simulink model "Roll_Pitch_LQIDG"  (R2020a)
settings: Solver=ode4  StartTime=0.0  StopTime=200  FixedStep=0.02  RelTol=1e-3
InitFcn:
  | LQIDG_solver;
values from neighbouring files (symbols this model uses):
  A1 = (h_cg * g * m_tot) / (m_tot * h_cg^2 + J_xx)    [QuadConstants.m]
  A3 = (b * d_cg) / (m_tot * h_cg^2 + J_xx)    [QuadConstants.m]
  A4 = (J_R) / (m_tot * h_cg^2 + J_xx)    [QuadConstants.m]
  A5 = (m1 * g * miu_k * r_x) / (m_tot * h_cg^2 + J_xx)    [QuadConstants.m]
  B3 = (b * d_cg) / (m_tot * h_cg^2 + J_yy)    [QuadConstants.m]
  LQIDG_openloop_pitch = (R1_inv * B' * p1)    [OpenLoop_LQDG_riccati_solver_pitch.m]
  LQIDG_openloop_roll = (R1_inv * B' * p1)    [OpenLoop_LQDG_riccati_solver_roll.m]
undefined symbols (not defined in the file or in its folder): A6, b, B6, d_cg, DiscIntNeverNeededParam, g, h_cg, J_R, J_yy, m2, m_tot, magnitude, miu_k, r_y
libraries: simulink x1, eeGeneralControl x1
settings Model: Creator=Ali  LastModifiedBy=Ali

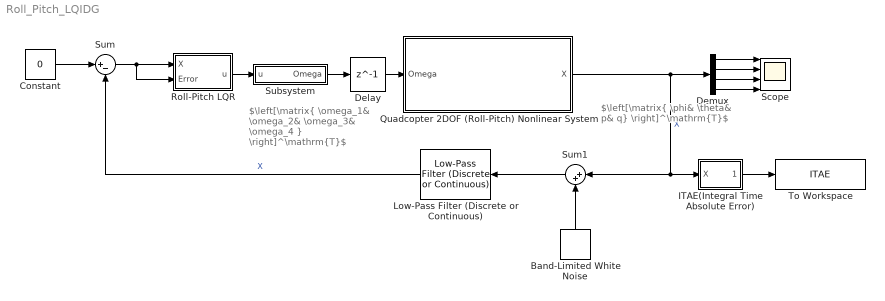
== system Roll_Pitch_LQIDG ==
  note: $\left[\matrix{ \omega_1& \omega_2& \omega_3& \omega_4 } \right]^\mathrm{T}$
  note: $\left[\matrix{ \phi& \theta& p& q} \right]^\mathrm{T}$
  Band-Limited White Noise : simulink/Sources/Band-Limited White Noise  Cov=[0.0001]  Ts=0.02  seed=[233419]
  Constant : Constant  Value=0
  Delay : Delay  DelayLength=1
  Demux : Demux
  ITAE(Integral Time Absolute Error) : Subsystem
  Low-Pass Filter (Discrete or Continuous) : eeGeneralControl/Low-Pass Filter (Discrete or Continuous)  K=1  T=0.05  B=inf  A=-inf  init_option=Inherited from block input  x0=0  Ts=-1
  Quadcopter 2DOF (Roll-Pitch) Nonlinear System : Subsystem  TreatAsAtomicUnit=on
  Roll-Pitch LQR : Subsystem
  Scope : Scope  NumInputPorts=4
  Subsystem : Subsystem
  Sum : Sum  Inputs=|+-
  Sum1 : Sum  Inputs=|++
  To Workspace : ToWorkspace  VariableName=ITAE  SaveFormat=Timeseries  SampleTime=-1
  wires:
  Subsystem/1(Omega) -> Delay/1
  Low-Pass Filter (Discrete or Continuous)/1 -> Sum/2  "X"
  Constant/1 -> Sum/1
  Sum/1 -> Roll-Pitch LQR/2(Error), Roll-Pitch LQR/1(X)
  Roll-Pitch LQR/1(u) -> Subsystem/1(u)
  Band-Limited White Noise/1 -> Sum1/2
  ITAE(Integral Time Absolute Error)/1(ITAE) -> To Workspace/1
  Quadcopter 2DOF (Roll-Pitch) Nonlinear System/1(X) -> Sum1/1, ITAE(Integral Time Absolute Error)/1(X), Demux/1  "X"
  Sum1/1 -> Low-Pass Filter (Discrete or Continuous)/1
  Demux/1 -> Scope/1
  Demux/2 -> Scope/2
  Demux/3 -> Scope/3
  Demux/4 -> Scope/4
  Delay/1 -> Quadcopter 2DOF (Roll-Pitch) Nonlinear System/1(Omega)

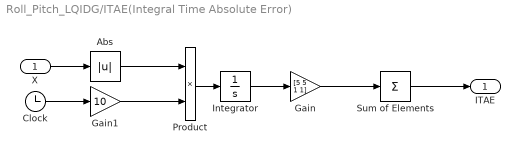
== system Roll_Pitch_LQIDG/ITAE(Integral Time Absolute Error) ==
  X : Inport
  Abs : Abs
  Clock : Clock
  Gain : Gain  Gain=[5 5 1 1]
  Gain1 : Gain  Gain=10
  Integrator : Integrator
  Product : Product
  Sum of Elements : Sum  Inputs=+
  ITAE : Outport
  wires:
  Product/1 -> Integrator/1
  Integrator/1 -> Gain/1
  Clock/1 -> Gain1/1
  Sum of Elements/1 -> ITAE/1
  Abs/1 -> Product/1
  X/1 -> Abs/1
  Gain/1 -> Sum of Elements/1
  Gain1/1 -> Product/2

== system Roll_Pitch_LQIDG/Quadcopter 2DOF (Roll-Pitch) Nonlinear System ==
  note: $\left[\matrix{ \phi& \theta& p& q} \right]^\mathrm{T}$
  note: $\left[\matrix{ \omega_1& \omega_2& \omega_3& \omega_4 } \right]^\mathrm{T}$
  note: $\left[\matrix{ \dot \phi& \dot \theta& \dot p& \dot q} \right]^\mathrm{T}$
  Omega : Inport
  For Each Subsystem : Subsystem  TreatAsAtomicUnit=on
  Integrator : Integrator  InitialCondition=[-0.1, -1, 0, 0]
  Quad System : Subsystem
  X : Outport
  wires:
  Integrator/1 -> Quad System/1(X), X/1  "X"
  Quad System/1(dot(X)) -> Integrator/1  "dot(X)"
  For Each Subsystem/1(Omega_m) -> Quad System/2(Omega)
  Omega/1 -> For Each Subsystem/1(Omega_c)

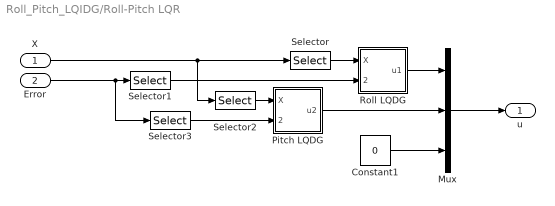
== system Roll_Pitch_LQIDG/Roll-Pitch LQR ==
  X : Inport
  Error : Inport  Port=2
  Constant1 : Constant  Value=0
  Mux : Mux  Inputs=3
  Pitch LQDG : Subsystem
  Roll LQDG : Subsystem
  Selector : Selector  InputPortWidth=4  IndexOptions=Index vector (dialog)  Indices=[1 3]  OutputSizes=1
  Selector1 : Selector  InputPortWidth=4  IndexOptions=Index vector (dialog)  Indices=[1 3]  OutputSizes=1
  Selector2 : Selector  InputPortWidth=4  IndexOptions=Index vector (dialog)  Indices=[2 4]  OutputSizes=1
  Selector3 : Selector  InputPortWidth=4  IndexOptions=Index vector (dialog)  Indices=[2 4]  OutputSizes=1
  u : Outport
  wires:
  Pitch LQDG/1(u2) -> Mux/2
  Roll LQDG/1(u1) -> Mux/1
  Constant1/1 -> Mux/3
  Mux/1 -> u/1
  X/1 -> Selector/1, Selector2/1
  Error/1 -> Selector3/1, Selector1/1
  Selector/1 -> Roll LQDG/1(X)
  Selector1/1 -> Roll LQDG/2(Error)
  Selector2/1 -> Pitch LQDG/1(X)
  Selector3/1 -> Pitch LQDG/2(Error)

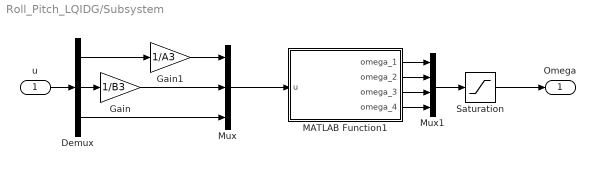
== system Roll_Pitch_LQIDG/Subsystem ==
  u : Inport
  Demux : Demux  Outputs=3
  Gain : Gain  Gain=1/B3
  Gain1 : Gain  Gain=1/A3
  MATLAB Function1 : MATLAB Function  TreatAsAtomicUnit=on
  Mux : Mux  Inputs=3
  Mux1 : Mux
  Saturation : Saturate  UpperLimit=6000/60*2*pi  LowerLimit=1300/60*2*pi
  Omega : Outport
  wires:
  MATLAB Function1/1(omega_1) -> Mux1/1
  MATLAB Function1/2(omega_2) -> Mux1/2
  MATLAB Function1/4(omega_4) -> Mux1/4
  Mux1/1 -> Saturation/1
  MATLAB Function1/3(omega_3) -> Mux1/3
  Saturation/1 -> Omega/1
  Mux/1 -> MATLAB Function1/1(u)
  Gain/1 -> Mux/2
  Gain1/1 -> Mux/1
  u/1 -> Demux/1
  Demux/2 -> Gain/1
  Demux/1 -> Gain1/1
  Demux/3 -> Mux/3

== system Roll_Pitch_LQIDG/Quadcopter 2DOF (Roll-Pitch) Nonlinear System/For Each Subsystem ==
  Omega_c : Inport  Partition=on  PartitionDimension=1  PartitionWidth=1  PartitionOffset=0
  Delay : Delay  DelayLength=1
  For Each : ForEach  DisableCoverage=on
  Transfer Fcn : TransferFcn  Denominator=[0.15 1]
  Omega_m : Outport  ConcatenationDimension=1
  wires:
  Delay/1 -> Transfer Fcn/1
  Omega_c/1 -> Delay/1
  Transfer Fcn/1 -> Omega_m/1

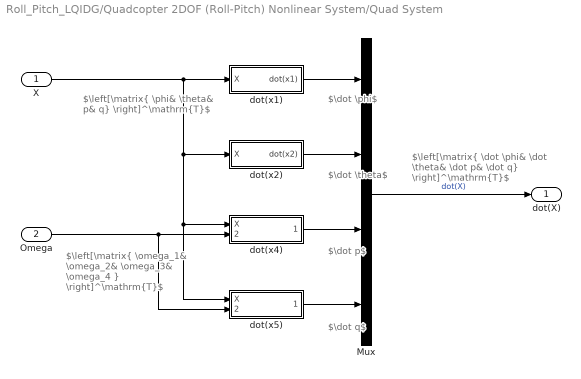
== system Roll_Pitch_LQIDG/Quadcopter 2DOF (Roll-Pitch) Nonlinear System/Quad System ==
  note: $\left[\matrix{ \omega_1& \omega_2& \omega_3& \omega_4 } \right]^\mathrm{T}$
  note: $\left[\matrix{ \phi& \theta& p& q} \right]^\mathrm{T}$
  note: $\left[\matrix{ \dot \phi& \dot \theta& \dot p& \dot q} \right]^\mathrm{T}$
  note: $\dot \phi$
  note: $\dot \theta$
  note: $\dot p$
  note: $\dot q$
  X : Inport
  Omega : Inport  Port=2
  Mux : Mux
  dot(x1) : Subsystem
  dot(x2) : Subsystem
  dot(x4) : Subsystem
  dot(x5) : Subsystem
  dot(X) : Outport
  wires:
  Mux/1 -> dot(X)/1  "dot(X)"
  X/1 -> dot(x5)/1(X), dot(x4)/1(X), dot(x2)/1(X), dot(x1)/1(X)
  Omega/1 -> dot(x5)/2(Omega), dot(x4)/2(Omega)
  dot(x5)/1(dot(x5)) -> Mux/4
  dot(x2)/1(dot(x2)) -> Mux/2
  dot(x1)/1(dot(x1)) -> Mux/1
  dot(x4)/1(dot(x4)) -> Mux/3

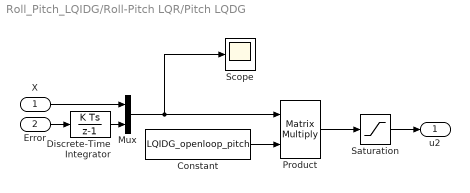
== system Roll_Pitch_LQIDG/Roll-Pitch LQR/Pitch LQDG ==
  X : Inport
  Error : Inport  Port=2
  Constant : Constant  Value=LQIDG_openloop_pitch
  Discrete-Time Integrator : DiscreteIntegrator  SampleTime=-1  LimitOutput=on  UpperSaturationLimit=5  LowerSaturationLimit=-5  ICPrevOutput=DiscIntNeverNeededParam  ICPrevScaledInput=DiscIntNeverNeededParam
  Mux : Mux  Inputs=2
  Product : Product  Multiplication=Matrix(*)
  Saturation : Saturate  UpperLimit=12  LowerLimit=-12
  Scope : Scope
  u2 : Outport
  wires:
  Product/1 -> Saturation/1
  Constant/1 -> Product/2
  X/1 -> Mux/1
  Mux/1 -> Scope/1, Product/1
  Saturation/1 -> u2/1
  Error/1 -> Discrete-Time Integrator/1
  Discrete-Time Integrator/1 -> Mux/2

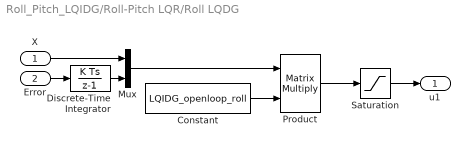
== system Roll_Pitch_LQIDG/Roll-Pitch LQR/Roll LQDG ==
  X : Inport
  Error : Inport  Port=2
  Constant : Constant  Value=LQIDG_openloop_roll
  Discrete-Time Integrator : DiscreteIntegrator  SampleTime=-1  LimitOutput=on  UpperSaturationLimit=5  LowerSaturationLimit=-5  ICPrevOutput=DiscIntNeverNeededParam  ICPrevScaledInput=DiscIntNeverNeededParam
  Mux : Mux  Inputs=2
  Product : Product  Multiplication=Matrix(*)
  Saturation : Saturate  UpperLimit=12  LowerLimit=-12
  u1 : Outport
  wires:
  Product/1 -> Saturation/1
  Constant/1 -> Product/2
  X/1 -> Mux/1
  Mux/1 -> Product/1
  Saturation/1 -> u1/1
  Error/1 -> Discrete-Time Integrator/1
  Discrete-Time Integrator/1 -> Mux/2

== system Roll_Pitch_LQIDG/Quadcopter 2DOF (Roll-Pitch) Nonlinear System/Quad System/dot(x1) ==
  X : Inport
  1 : Subsystem
  Add : Sum
  Subsystem1 : Subsystem
  dot(x1) : Outport
  wires:
  X/1 -> Subsystem1/1(X), 1/1(X)  "X"
  Subsystem1/1(x4) -> Add/2
  Add/1 -> dot(x1)/1
  1/1(x5sin(x1)tan(x2)) -> Add/1

== system Roll_Pitch_LQIDG/Quadcopter 2DOF (Roll-Pitch) Nonlinear System/Quad System/dot(x2) ==
  X : Inport
  1 : Subsystem
  dot(x2) : Outport
  wires:
  X/1 -> 1/1(X)  "X"
  1/1(x5cos(x1)) -> dot(x2)/1

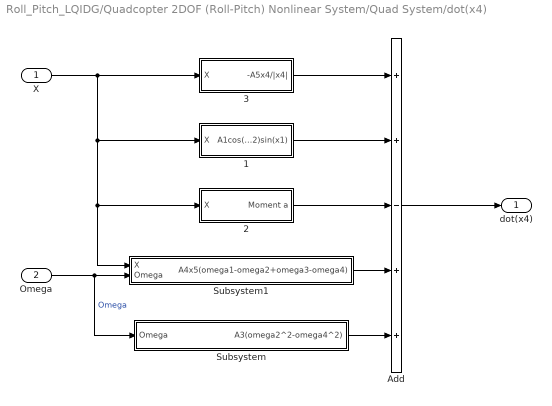
== system Roll_Pitch_LQIDG/Quadcopter 2DOF (Roll-Pitch) Nonlinear System/Quad System/dot(x4) ==
  X : Inport
  Omega : Inport  Port=2
  1 : Subsystem
  2 : Subsystem
  3 : Subsystem
  Add : Sum  Inputs=++-++
  Subsystem : Subsystem
  Subsystem1 : Subsystem
  dot(x4) : Outport
  wires:
  X/1 -> 2/1(X), Subsystem1/1(X), 1/1(X), 3/1(X)
  Omega/1 -> Subsystem/1(Omega), Subsystem1/2(Omega)  "Omega"
  Add/1 -> dot(x4)/1
  3/1("-A5x4/|x4| ") -> Add/1
  1/1(A1cos(x2)sin(x1)) -> Add/2
  Subsystem1/1(A4x5(omega1-omega2+omega3-omega4)) -> Add/4
  Subsystem/1(A3(omega2^2-omega4^2)) -> Add/5
  2/1(Moment a) -> Add/3

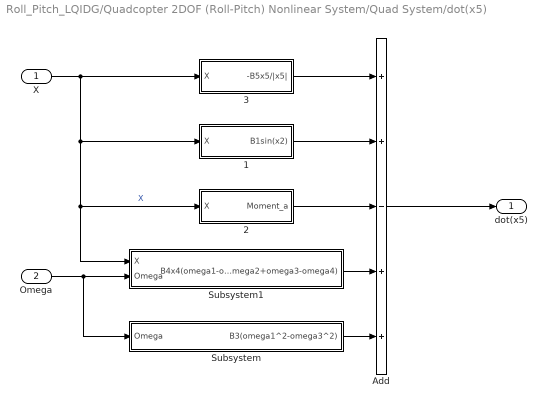
== system Roll_Pitch_LQIDG/Quadcopter 2DOF (Roll-Pitch) Nonlinear System/Quad System/dot(x5) ==
  X : Inport
  Omega : Inport  Port=2
  1 : Subsystem
  2 : Subsystem
  3 : Subsystem
  Add : Sum  Inputs=++-++
  Subsystem : Subsystem
  Subsystem1 : Subsystem
  dot(x5) : Outport
  wires:
  Omega/1 -> Subsystem/1(Omega), Subsystem1/2(Omega)
  Add/1 -> dot(x5)/1
  3/1("-B5x5/|x5| ") -> Add/1
  1/1(B1sin(x2)) -> Add/2
  X/1 -> 2/1(X), Subsystem1/1(X), 1/1(X), 3/1(X)  "X"
  Subsystem/1(B3(omega1^2-omega3^2)) -> Add/5
  Subsystem1/1(B4x4(omega1-omega2+omega3-omega4)) -> Add/4
  2/1(Moment_a) -> Add/3

== system Roll_Pitch_LQIDG/Quadcopter 2DOF (Roll-Pitch) Nonlinear System/Quad System/dot(x1)/1 ==
  X : Inport
  Demux : Demux  Outputs=3
  Selector : Selector  InputPortWidth=4  IndexOptions=Index vector (dialog)  Indices=[1 2 4]  OutputSizes=1
  Subsystem : Subsystem
  x5sin(x1)tan(x2) : Outport
  wires:
  Demux/2 -> Subsystem/2(x2)  "x2"
  X/1 -> Selector/1  "x"
  Demux/1 -> Subsystem/1(x1)  "x1"
  Demux/3 -> Subsystem/3(x5)  "x5"
  Subsystem/1(x5sin(x1)tan(x2)) -> x5sin(x1)tan(x2)/1
  Selector/1 -> Demux/1

== system Roll_Pitch_LQIDG/Quadcopter 2DOF (Roll-Pitch) Nonlinear System/Quad System/dot(x1)/Subsystem1 ==
  X : Inport
  Selector : Selector  InputPortWidth=4  IndexOptions=Index vector (dialog)  Indices=[3]  OutputSizes=1
  x4 : Outport
  wires:
  Selector/1 -> x4/1
  X/1 -> Selector/1

== system Roll_Pitch_LQIDG/Quadcopter 2DOF (Roll-Pitch) Nonlinear System/Quad System/dot(x2)/1 ==
  X : Inport
  Demux : Demux  Outputs=2
  Selector : Selector  InputPortWidth=4  IndexOptions=Index vector (dialog)  Indices=[1 4]  OutputSizes=1
  Subsystem : Subsystem
  x5cos(x1) : Outport
  wires:
  X/1 -> Selector/1  "x"
  Demux/1 -> Subsystem/1(x1)  "x1"
  Demux/2 -> Subsystem/2(x5)  "x5"
  Subsystem/1(Out1) -> x5cos(x1)/1
  Selector/1 -> Demux/1

== system Roll_Pitch_LQIDG/Quadcopter 2DOF (Roll-Pitch) Nonlinear System/Quad System/dot(x4)/1 ==
  X : Inport
  Demux : Demux  Outputs=2
  Selector : Selector  InputPortWidth=4  IndexOptions=Index vector (dialog)  Indices=[1 2]  OutputSizes=1
  Subsystem : Subsystem
  A1cos(x2)sin(x1) : Outport
  wires:
  Demux/1 -> Subsystem/1(x1)  "x1"
  Subsystem/1(A1cos(x2)sin(x1)) -> A1cos(x2)sin(x1)/1
  Demux/2 -> Subsystem/2(x2)  "x2"
  X/1 -> Selector/1  "x"
  Selector/1 -> Demux/1

== system Roll_Pitch_LQIDG/Quadcopter 2DOF (Roll-Pitch) Nonlinear System/Quad System/dot(x4)/2 ==
  X : Inport
  Selector : Selector  InputPortWidth=4  IndexOptions=Index vector (dialog)  Indices=[1]  OutputSizes=1
  Subsystem : Subsystem
  Moment a : Outport
  wires:
  Selector/1 -> Subsystem/1(x1)  "x1"
  Subsystem/1(Moment_a) -> Moment a/1
  X/1 -> Selector/1  "x"

== system Roll_Pitch_LQIDG/Quadcopter 2DOF (Roll-Pitch) Nonlinear System/Quad System/dot(x4)/3 ==
  X : Inport
  Selector : Selector  InputPortWidth=4  IndexOptions=Index vector (dialog)  Indices=[3]  OutputSizes=1
  Subsystem : Subsystem
  "-A5x4/|x4| " : Outport
  wires:
  Subsystem/1("-A5x4/|x4| ") -> "-A5x4/|x4| "/1
  Selector/1 -> Subsystem/1(x4)
  X/1 -> Selector/1  "x"

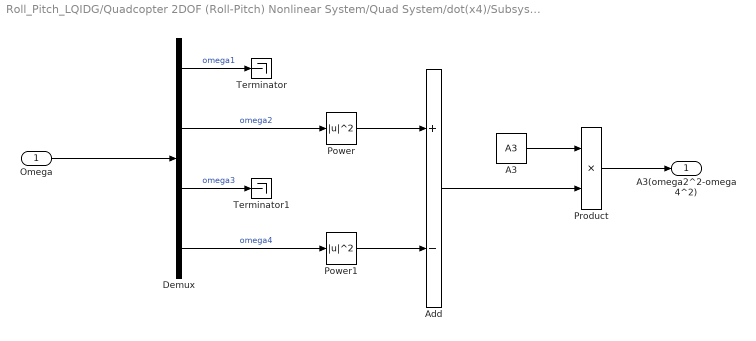
== system Roll_Pitch_LQIDG/Quadcopter 2DOF (Roll-Pitch) Nonlinear System/Quad System/dot(x4)/Subsystem ==
  Omega : Inport
  A3 : Constant  Value=A3
  Add : Sum  Inputs=+-
  Demux : Demux
  Power : Math  Operator=magnitude^2  SaturateOnIntegerOverflow=on
  Power1 : Math  Operator=magnitude^2  SaturateOnIntegerOverflow=on
  Product : Product
  Terminator : Terminator
  Terminator1 : Terminator
  A3(omega2^2-omega4^2) : Outport
  wires:
  Product/1 -> A3(omega2^2-omega4^2)/1
  Power1/1 -> Add/2
  Demux/2 -> Power/1  "omega2"
  Demux/4 -> Power1/1  "omega4"
  Add/1 -> Product/2
  Power/1 -> Add/1
  A3/1 -> Product/1
  Omega/1 -> Demux/1
  Demux/3 -> Terminator1/1  "omega3"
  Demux/1 -> Terminator/1  "omega1"

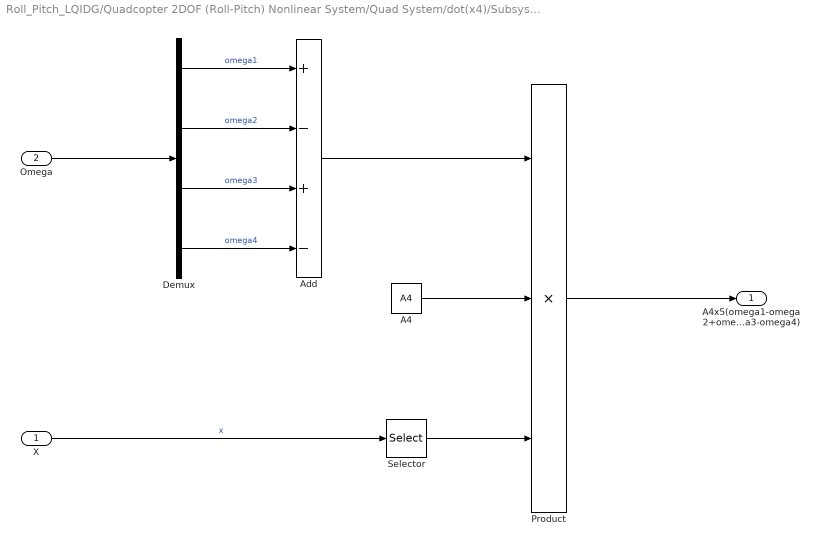
== system Roll_Pitch_LQIDG/Quadcopter 2DOF (Roll-Pitch) Nonlinear System/Quad System/dot(x4)/Subsystem1 ==
  X : Inport
  Omega : Inport  Port=2
  A4 : Constant  Value=A4
  Add : Sum  Inputs=+-+-
  Demux : Demux
  Product : Product  Inputs=3
  Selector : Selector  InputPortWidth=4  IndexOptions=Index vector (dialog)  Indices=[4]  OutputSizes=1
  A4x5(omega1-omega2+omega3-omega4) : Outport
  wires:
  Omega/1 -> Demux/1
  Demux/1 -> Add/1  "omega1"
  Demux/2 -> Add/2  "omega2"
  Demux/3 -> Add/3  "omega3"
  Demux/4 -> Add/4  "omega4"
  Add/1 -> Product/1
  A4/1 -> Product/2
  Product/1 -> A4x5(omega1-omega2+omega3-omega4)/1
  Selector/1 -> Product/3
  X/1 -> Selector/1  "x"

== system Roll_Pitch_LQIDG/Quadcopter 2DOF (Roll-Pitch) Nonlinear System/Quad System/dot(x5)/1 ==
  X : Inport
  Selector : Selector  InputPortWidth=4  IndexOptions=Index vector (dialog)  Indices=[2]  OutputSizes=1
  Subsystem : Subsystem
  B1sin(x2) : Outport
  wires:
  Subsystem/1(B1sin(x2)) -> B1sin(x2)/1
  Selector/1 -> Subsystem/1(x2)
  X/1 -> Selector/1  "x"

== system Roll_Pitch_LQIDG/Quadcopter 2DOF (Roll-Pitch) Nonlinear System/Quad System/dot(x5)/2 ==
  X : Inport
  Selector : Selector  InputPortWidth=4  IndexOptions=Index vector (dialog)  Indices=[2]  OutputSizes=1
  Subsystem : Subsystem
  Moment_a : Outport
  wires:
  X/1 -> Selector/1  "x"
  Subsystem/1(moment_a) -> Moment_a/1
  Selector/1 -> Subsystem/1(In1)

== system Roll_Pitch_LQIDG/Quadcopter 2DOF (Roll-Pitch) Nonlinear System/Quad System/dot(x5)/3 ==
  X : Inport
  Selector : Selector  InputPortWidth=4  IndexOptions=Index vector (dialog)  Indices=[4]  OutputSizes=1
  Subsystem : Subsystem
  "-B5x5/|x5| " : Outport
  wires:
  Selector/1 -> Subsystem/1(x5)  "x5"
  Subsystem/1("-B5x5/|x5| ") -> "-B5x5/|x5| "/1
  X/1 -> Selector/1  "x"

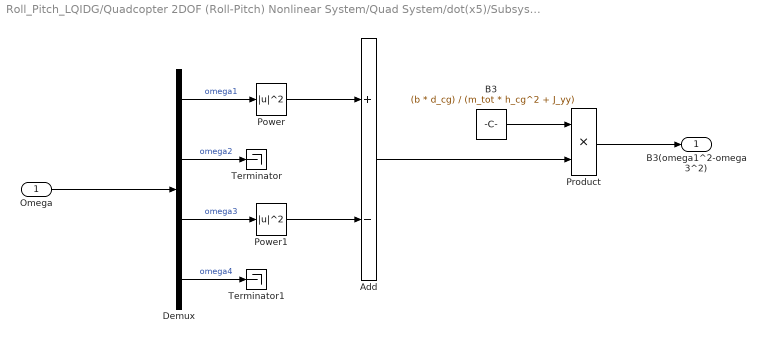
== system Roll_Pitch_LQIDG/Quadcopter 2DOF (Roll-Pitch) Nonlinear System/Quad System/dot(x5)/Subsystem ==
  Omega : Inport
  Add : Sum  Inputs=+-
  B3 : Constant  Value=(b * d_cg) / (m_tot * h_cg^2 + J_yy)
  Demux : Demux
  Power : Math  Operator=magnitude^2  SaturateOnIntegerOverflow=on
  Power1 : Math  Operator=magnitude^2  SaturateOnIntegerOverflow=on
  Product : Product
  Terminator : Terminator
  Terminator1 : Terminator
  B3(omega1^2-omega3^2) : Outport
  wires:
  Product/1 -> B3(omega1^2-omega3^2)/1
  Power1/1 -> Add/2
  Add/1 -> Product/2
  Power/1 -> Add/1
  B3/1 -> Product/1
  Omega/1 -> Demux/1
  Demux/3 -> Power1/1  "omega3"
  Demux/1 -> Power/1  "omega1"
  Demux/2 -> Terminator/1  "omega2"
  Demux/4 -> Terminator1/1  "omega4"

== system Roll_Pitch_LQIDG/Quadcopter 2DOF (Roll-Pitch) Nonlinear System/Quad System/dot(x5)/Subsystem1 ==
  X : Inport
  Omega : Inport  Port=2
  Add : Sum  Inputs=+-+-
  B4 : Constant  Value=(-J_R) / (m_tot * h_cg^2 + J_yy)
  Demux : Demux
  Product : Product  Inputs=3
  Selector : Selector  InputPortWidth=4  IndexOptions=Index vector (dialog)  Indices=[3]  OutputSizes=1
  B4x4(omega1-omega2+omega3-omega4) : Outport
  wires:
  Omega/1 -> Demux/1
  Demux/1 -> Add/1  "omega1"
  Demux/2 -> Add/2  "omega2"
  Demux/3 -> Add/3  "omega3"
  Demux/4 -> Add/4  "omega4"
  Add/1 -> Product/1
  B4/1 -> Product/2
  Product/1 -> B4x4(omega1-omega2+omega3-omega4)/1
  Selector/1 -> Product/3
  X/1 -> Selector/1  "x"

== system Roll_Pitch_LQIDG/Quadcopter 2DOF (Roll-Pitch) Nonlinear System/Quad System/dot(x1)/1/Subsystem ==
  x1 : Inport
  x2 : Inport  Port=2
  x5 : Inport  Port=3
  Product : Product  Inputs=3
  Sin : Trigonometry
  Tan : Trigonometry  Operator=tan
  x5sin(x1)tan(x2) : Outport
  wires:
  Sin/1 -> Product/1
  x5/1 -> Product/3
  Product/1 -> x5sin(x1)tan(x2)/1
  x1/1 -> Sin/1
  x2/1 -> Tan/1
  Tan/1 -> Product/2

== system Roll_Pitch_LQIDG/Quadcopter 2DOF (Roll-Pitch) Nonlinear System/Quad System/dot(x2)/1/Subsystem ==
  x1 : Inport
  x5 : Inport  Port=2
  Cos : Trigonometry  Operator=cos
  Product : Product
  Out1 : Outport
  wires:
  Cos/1 -> Product/1
  Product/1 -> Out1/1
  x1/1 -> Cos/1
  x5/1 -> Product/2

== system Roll_Pitch_LQIDG/Quadcopter 2DOF (Roll-Pitch) Nonlinear System/Quad System/dot(x4)/1/Subsystem ==
  x1 : Inport
  x2 : Inport  Port=2
  A1 : Constant  Value=A1
  Cos : Trigonometry  Operator=cos
  Product : Product  Inputs=3
  Sin : Trigonometry
  A1cos(x2)sin(x1) : Outport
  wires:
  Sin/1 -> Product/1
  Product/1 -> A1cos(x2)sin(x1)/1
  x1/1 -> Sin/1
  x2/1 -> Cos/1
  Cos/1 -> Product/2
  A1/1 -> Product/3

== system Roll_Pitch_LQIDG/Quadcopter 2DOF (Roll-Pitch) Nonlinear System/Quad System/dot(x4)/2/Subsystem ==
  x1 : Inport
  A6 : Constant  Value=A6
  Product : Product
  Sin : Trigonometry  Operator=cos
  Moment_a : Outport
  wires:
  Sin/1 -> Product/1
  Product/1 -> Moment_a/1
  x1/1 -> Sin/1
  A6/1 -> Product/2

== system Roll_Pitch_LQIDG/Quadcopter 2DOF (Roll-Pitch) Nonlinear System/Quad System/dot(x4)/3/Subsystem ==
  x4 : Inport
  A5 : Constant  Value=A5
  Gain : Gain  Gain=-1
  Switch : Switch  Criteria=u2 > Threshold
  "-A5x4/|x4| " : Outport
  wires:
  Switch/1 -> "-A5x4/|x4| "/1
  A5/1 -> Switch/3, Gain/1
  x4/1 -> Switch/2
  Gain/1 -> Switch/1

== system Roll_Pitch_LQIDG/Quadcopter 2DOF (Roll-Pitch) Nonlinear System/Quad System/dot(x5)/1/Subsystem ==
  x2 : Inport
  B1 : Constant  Value=(h_cg * g * m_tot) / (m_tot * h_cg^2 + J_yy)
  Product : Product
  Sin : Trigonometry
  B1sin(x2) : Outport
  wires:
  Product/1 -> B1sin(x2)/1
  x2/1 -> Sin/1
  B1/1 -> Product/2
  Sin/1 -> Product/1

== system Roll_Pitch_LQIDG/Quadcopter 2DOF (Roll-Pitch) Nonlinear System/Quad System/dot(x5)/2/Subsystem ==
  In1 : Inport
  B6 : Constant  Value=B6
  Cos : Trigonometry  Operator=cos
  Product : Product
  moment_a : Outport
  wires:
  Product/1 -> moment_a/1
  B6/1 -> Product/1
  In1/1 -> Cos/1
  Cos/1 -> Product/2

== system Roll_Pitch_LQIDG/Quadcopter 2DOF (Roll-Pitch) Nonlinear System/Quad System/dot(x5)/3/Subsystem ==
  x5 : Inport
  B5 : Constant  Value=(m2 * g * miu_k * r_y) / (m_tot * h_cg^2 + J_yy)
  Gain : Gain  Gain=-1
  Switch : Switch  Criteria=u2 > Threshold
  "-B5x5/|x5| " : Outport
  wires:
  Switch/1 -> "-B5x5/|x5| "/1
  B5/1 -> Switch/3, Gain/1
  x5/1 -> Switch/2
  Gain/1 -> Switch/1

== matlab function Roll_Pitch_LQIDG/Subsystem/MATLAB Function1 ==
  data: u input size=3; omega_1 output size=1; omega_2 output size=1; omega_3 output size=1; omega_4 output size=1
function [omega_1, omega_2, omega_3, omega_4] = fcn(u)
u1 = u(1);
u2 = u(2);
u3 = u(3);
% control effort
u4 = ones(1, length(u1)) * 4 * rpm2rad_sec(2000)^2;
% calculate omega
if (u4 + u3 + 2 * u2) / 4 > 0
    omega_1 = sqrt((u4 + u3 + 2 * u2) / 4);
else
    omega_1 = 0;
end
if (u4 + u3 - 2 * u2) / 4 > 0
    omega_3 = sqrt((u4 + u3 - 2 * u2) / 4);
else
    omega_3 = 0;
end
if (u4 - u3 + 2 * u1) / 4 > 0
    omega_2 = sqrt((u4 - u3 + 2 * u1) / 4);
else
    omega_2 = 0;
end
if (u4 - u3 - 2 * u1) / 4 > 0
    omega_4 = sqrt((u4 - u3 - 2 * u1) / 4);
else
    omega_4 = 0;
end
end
%% functions
% rpm to rad/sec
function rad = rpm2rad_sec(rpm)
rad = rpm / 60 * 2 * pi;
end
